simulink model "EVCS_model_v2"  (R2024b)
settings: Solver=VariableStepAuto  StartTime=0.0  StopTime=210  MaxStep=1e-3  RelTol=1e-2  AbsTol=1e-3
undefined symbols (not defined in the file or in its folder): FC, gcbh, Ion, Lithium, P, sps_rtmsupport, Ts
libraries: spsSeriesRLCBranchLib x40, spsIGBTDiodeLib x8, slpidlib x7, spsVoltageMeasurementLib x7, spsCurrentMeasurementLib x6, eeGeneralControl x4, spsMosfetLib x4, spsPWMGeneratorDCDCLib x3, spsAlphaBetaZerotodq0Lib x2, spsBatteryLib x2, spsDiodeLib x2, spsBreakerLib x1
(part 1 of 2)
settings Model: Creator=VidhiGupta  LastModifiedBy=akshat
settings RTWCC: GPUComputeCapability=3.5

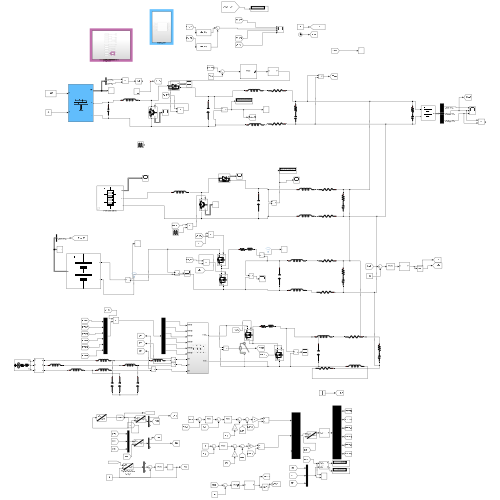
[thumbnail: Simulink's stored preview of the top-level diagram]
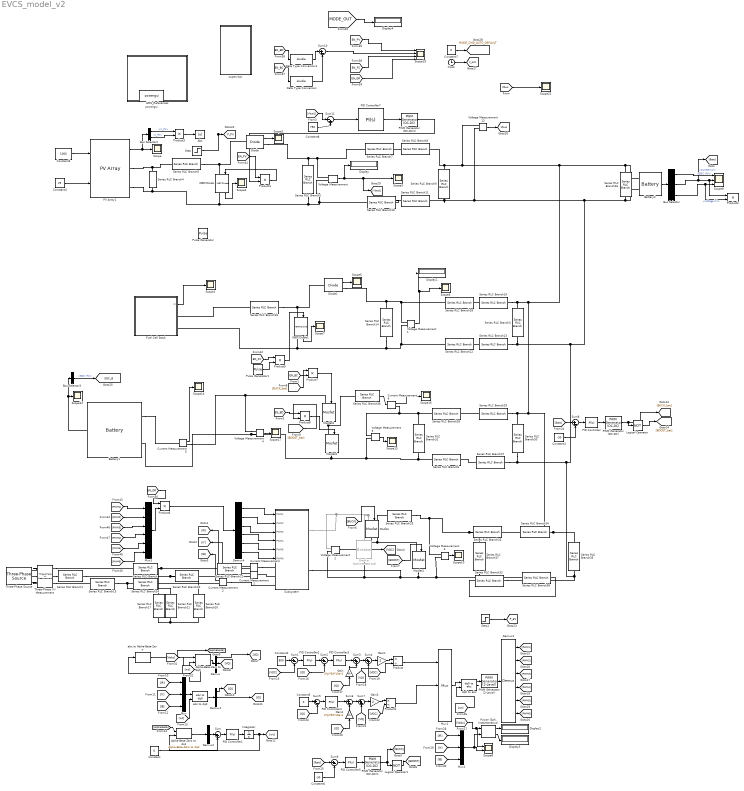
== system EVCS_model_v2 ==
  Abs : Abs  SaturateOnIntegerOverflow=off
  Alpha-Beta-Zero to dq0 : spsAlphaBetaZerotodq0Lib/Alpha-Beta-Zero to dq0  Alignment=90 degrees behind phase A axis
  Alpha-Beta-Zero to dq1 : spsAlphaBetaZerotodq0Lib/Alpha-Beta-Zero to dq0  Alignment=90 degrees behind phase A axis
  Battery1 : spsBatteryLib/Battery  BatType=Lithium-Ion  NomV=400  NomQ=250  SOC=60  Batt_Tr=30  PresetModel=on  MaxQ=250  MinV=300  FullV=465.5949  Dis_rate=108.6957  R=0.016  Normal_OP=226.087  expZone="[432.1543      12.28261]"
  Battery2 : spsBatteryLib/Battery  BatType=Lithium-Ion  NomV=400  NomQ=188  SOC=30  Batt_Tr=1  PresetModel=on  MaxQ=188  MinV=300  FullV=465.5949  Dis_rate=81.7391  R=0.021277  Normal_OP=170.0174  expZone="[432.1543      9.236522]"
  Breaker : spsBreakerLib/Breaker  Commented=on  InitialState=0  SwitchingTimes="[1/60  5/60]"  External=off  BreakerResistance=0.000001  SnubberResistance=1e6  SnubberCapacitance=inf  Measurements=None  MoreParameters=on  NoBreakLoop=off
  Bus Selector : BusSelector  OutputSignals=SOC (%),Current (A),Voltage (V)
  Bus Selector2 : BusSelector  OutputSignals=V_PV,I_PV
  Bus Selector3 : BusSelector  OutputSignals=SOC (%)
  Clock : Clock
  Constant : Constant  Value=0
  Constant1 : Constant  Value=-30
  Constant2 : Constant  Value=800
  Constant3 : Constant  Value=1000
  Constant4 : Constant  Value=25
  Constant5 : Constant  Value=0
  Constant6 : Constant  Value=-30
  Constant7 : Constant  Value=0
  Constant8 : Constant  Value=750
  Current Measurement{,1..2,5..6} (5 alike) : spsCurrentMeasurementLib/Current Measurement  PhasorSimulation=off  OutputType=Complex  PSBequivalent=0
  Data Type Conversion : DataTypeConversion  OutDataTypeStr=double  SaturateOnIntegerOverflow=off  RndMeth=Floor
  Data Type Conversion1 : DataTypeConversion  OutDataTypeStr=double  SaturateOnIntegerOverflow=off  RndMeth=Floor
  Demux : Demux  Outputs=3
  Demux1 : Demux  Outputs=3
  Demux2 : Demux  Outputs=3
  Demux3 : Demux  Outputs=6
  Demux4 : Demux  Outputs=6
  Diode : spsDiodeLib/Diode  Ron=0.001  Lon=0  Vf=0.8  IC=0  UseSnubber=0  Rs=500  Cs=250e-9  Measurements=on
  Diode1 : spsDiodeLib/Diode  Ron=0.001  Lon=0  Vf=0.8  IC=0  UseSnubber=0  Rs=500  Cs=250e-9  Measurements=on
  Display{,1..4} (5 alike) : Display
  EMS_References : Subsystem
  Fuel Cell Stack : Subsystem  AncestorBlock=sps_lib/Sources/Fuel Cell Stack  LoadFcn=sps_rtmsupport('LoadFcn',gcbh);  StartFcn=sps_rtmsupport('StartFcn',gcbh);  StopFcn=sps_rtmsupport('StopFcn',gcbh);  mask(Fuel Cell Stack){PresetModel=No (User-Defined), FcType=0, Detailed=Simplified, Eoc=P.FC.Eoc, NomVI=P.FC.NomVI, EndVI=P.FC.EndVI, Nc=P.FC.Nc, n=55, TOp=65, AirFr=2500, SuppPress=[3, 1.5], Comp=[99.95,21,1], SignX=off, SignY=off, FlowRateH2=off, FlowRateAir=off, SystemTemp=off, SystemPH2=off, SystemPAir=off, FCDyn=off, FC_tau=1, Peak_O2=80, V_Under=10}
      mask prompts: PresetModel "Preset model:"; FcType "Fuel Cell type:"; Detailed "Model detail Level:"; Eoc "Voltage at 0A and 1A [V_0(V), V_1(V)]"; NomVI "Nominal operating point [Inom(A), Vnom(V)]"; EndVI "Maximum operating point [Iend(A), Vend(V)]"; Nc "Number of cells"; n "Nominal stack efficiency (%)"; TOp "Operating temperature (Celsius)"; AirFr "Nominal Air flow rate (lpm)"; SuppPress "Nominal supply pressure [Fuel (atm), Air (atm)]"; Comp "Nominal composition (%) [H2 O2 H2O(Air)]"; SignX "Fuel  composition [x_H2(%)]"; SignY "Oxidant composition [y_O2(%)]"; FlowRateH2 "Fuel flow rate [FuelFr(lpm)]"; FlowRateAir "Air flow rate [AirFr(lpm)]"; SystemTemp "System Temperature [T(Kelvin)]"; SystemPH2 "Fuel supply pressure [Pfuel(bar)]"; SystemPAir "Air supply pressure [PAir(bar)]"; FCDyn "Specify Fuel Cell Dynamics?"; FC_tau "Fuel Cell response time (sec)"; Peak_O2 "Peak O2 utilization (%)"; V_Under "Voltage undershoot (V) @ peak O2 utilization"
      mask help:
      | Implements a generic hydrogen fuel cell model which allows the simulation for the following types of cells:
      | - Proton Exchange Membrane Fuel Cell (PEMFC)
      | - Solid Oxide Fuel Cell (SOFC)
      | - Alkaline Fuel Cell (AFC)
      mask init:
      | block = gcb;
      | %% DO NOT CHANGE THIS ORDER
      | FuelCellBlockCback(block,'Inputs')
      | [FC, WantBlockChoice, Ts] = FuelCellBlockInit(block,Eoc,NomVI,EndVI,Nc,n,TOp,AirFr,SuppPress,Comp,FlowRateH2,FlowRateAir);
      | powericon('SetInternalModels','set',block,WantBlockChoice);
      settings: LibrarySourceBlock=sps_lib/Sources/Fuel Cell Stack  CopyFcn=sps_rtmsupport('CopyFcn',gcbh);  DeleteFcn=sps_rtmsupport('DeleteFcn',gcbh);  UndoDeleteFcn=sps_rtmsupport('UndoDeleteFcn',gcbh);  ModelCloseFcn=sps_rtmsupport('ModelCloseFcn',gcbh);  PreSaveFcn=sps_rtmsupport('PreSaveFcn',gcbh);  PostSaveFcn=sps_rtmsupport('PostSaveFcn',gcbh);  NameChangeFcn=sps_rtmsupport('NameChangeFcn',gcbh);  PreCopyFcn=sps_rtmsupport('PreCopyFcn',gcbh);  OpenFcn=sps_rtmsupport('OpenFcn',gcbh, [1 2 3 13 14 15 16 17 18 19 20]);  CloseFcn=sps_rtmsupport('CloseFcn',gcbh);  PreDeleteFcn=sps_rtmsupport('PreDeleteFcn',gcbh);
      mask Help: helpview(psbhelp)
      mask TypeOptions PresetModel: No (User-Defined) | PEMFC - 1.26 kW - 24 Vdc | PEMFC - 6 kW - 45 Vdc | PEMFC - 50 kW - 625 Vdc | AFC - 2.4 kW - 48 Vdc | SOFC - 3 kW - 100 Vdc | SOFC - 25 kW - 630 Vdc
      mask Callback PresetModel: FuelCellBlockCback(gcb,'Preset')
      mask TypeOptions Detailed: Simplified | Detailed
      mask Callback Detailed: FuelCellBlockCback(gcb,'Visibilities')
      mask Callback FlowRateAir: FuelCellBlockCback(gcb,'Visibilities')
      mask Callback FCDyn: FuelCellBlockCback(gcb,'Visibilities')
      mask DialogControl ParameterTabVar0 Prompt: Parameters
      mask DialogControl plot_graph Prompt: Plot V_I characteristic
      mask DialogControl plot_graph Callback: FuelCellBlockCback(gcb,'PlotGraph');
      mask DialogControl ViewParam Prompt: View Cell parameters
      mask DialogControl ViewParam Callback: FuelCellBlockCback(gcb,'ViewParam');
      mask DialogControl ParameterTabVar01 Prompt: Signal variation
      mask DialogControl ParameterTabVar012 Prompt: Fuel Cell Dynamics
      mask Display: image(fullfile(matlabroot,'toolbox','physmod','powersys','library','sources','FuelCellStackBlockIcon.png'), [3,0,3,0,100,100]);
  Gain : Gain  Gain=2*pi*50*10e-3
  Gain1 : Gain  Gain=2
  Gain2 : Gain  Gain=2*pi*50*10e-3
  Gain3 : Gain  Gain=2
  IGBT/Diode : spsIGBTDiodeLib/IGBT//Diode  Ron=1e-3  Rs=1e5  Cs=inf  Measurements=on
  IGBT/Diode1 : spsIGBTDiodeLib/IGBT//Diode  Ron=1e-3  Rs=1e5  Cs=inf  Measurements=on
  Integrator : Integrator
  Logical Operator : Logic  Operator=NOT  AllPortsSameDT=off  OutDataTypeStr=boolean
  Logical Operator1 : Logic  Operator=NOT  AllPortsSameDT=off  OutDataTypeStr=boolean
  Mosfet{,1,3..4} (4 alike) : spsMosfetLib/Mosfet  Ron=0.001  Lon=0  Rd=1e-3  Vfd=0  IC=0  Rs=1e5  Cs=inf  Measurements=off
  Mux : Mux  Inputs=3
  Mux1 : Mux  Inputs=3
  Mux2 : Mux  Inputs=3
  Mux3 : Mux  Inputs=6
  PID Controller{,1..4} (5 alike) : slpidlib/PID Controller  Controller=PI  Form=Parallel  TimeDomain=Continuous-time  UseExternalTs=off  SampleTime=-1  IntegratorMethod=Forward Euler  FilterMethod=Forward Euler  ControllerParametersSource=internal  P=0.5  I=50  UseKiTs=off  D=0  UseExternalDerivativeSource=off  N=100  UseFilter=on  TunerSelectOption=Transfer Function Based (PID Tuner App)  InitialConditionSource=internal  InitialConditionForIntegrator=0  InitialConditionForFilter=0  DifferentiatorICPrevScaledInput=0  ExternalReset=none  TrackingMode=off  Kt=1  LimitOutput=off  SatLimitsSource=internal  UpperSaturationLimit=inf  LowerSaturationLimit=-inf  LinearizeAsGain=on  AntiWindupMode=none  Kb=1  LimitIntegrator=off  UpperIntegratorSaturationLimit=inf  LowerIntegratorSaturationLimit=-inf  POutMin=[]  POutMax=[]  IOutMin=[]  IOutMax=[]  DOutMin=[]  DOutMax=[]  NOutMin=[]  NOutMax=[]  SumOutMin=[]  SumOutMax=[]  SaturationOutMin=[]  SaturationOutMax=[]  PParamMin=[]  PParamMax=[]  IParamMin=[]  IParamMax=[]  DParamMin=[]  DParamMax=[]  NParamMin=[]  NParamMax=[]  KbParamMin=[]  KbParamMax=[]  KtParamMin=[]  KtParamMax=[]  KbOutMin=[]  KbOutMax=[]  KtOutMin=[]  KtOutMax=[]  IntegratorOutMin=[]  IntegratorOutMax=[]  FilterOutMin=[]  FilterOutMax=[]  SumI1OutMin=[]  SumI1OutMax=[]  SumI2OutMin=[]  SumI2OutMax=[]  SumI3OutMin=[]  SumI3OutMax=[]  SumI4OutMin=[]  SumI4OutMax=[]  SumDOutMin=[]  SumDOutMax=[]  DifferentiatorOutMin=[]  DifferentiatorOutMax=[]  FilterDiffOutCoefMin=[]  FilterDiffOutCoefMax=[]  ReciprocalOutMin=[]  ReciprocalOutMax=[]  SumDenOutMin=[]  SumDenOutMax=[]  SumNumOutMin=[]  SumNumOutMax=[]  DivideOutMin=[]  DivideOutMax=[]  UdiffTsProdOutMin=[]  UdiffTsProdOutMax=[]  NTsProdOutMin=[]  NTsProdOutMax=[]  UintegralTsProdOutMin=[]  UintegralTsProdOutMax=[]  UngainTsProdOutMin=[]  UngainTsProdOutMax=[]  ClampingZeroOutDataTypeStr=Inherit: Inherit via back propagation  ClampingZeroOutMin=[]  ClampingZeroOutMax=[]  FilterDenConstantOutDataTypeStr=Inherit: Inherit via back propagation  FilterDenConstantOutMin=[]  FilterDenConstantOutMax=[]  PCopyOutDataTypeStr=Inherit: Inherit via back propagation  PCopyOutMin=[]  PCopyOutMax=[]  NCopyOutDataTypeStr=Inherit: Inherit via back propagation  NCopyOutMin=[]  NCopyOutMax=[]  IntegratorContinuousStateAttributes=''  IntegratorStateMustResolveToSignalObject=off  IntegratorRTWStateStorageClass=Auto  FilterContinuousStateAttributes=''  FilterStateMustResolveToSignalObject=off  FilterRTWStateStorageClass=Auto  ParallelPVariant=InternalParameters  IdealPVariant=Disabled  IVariant=InternalParameters  DVariant=Disabled  IntegratorVariant=Continuous  SatVariant=Disabled  AWVariant=Passthrough  PCopyVariant=Disabled  TRVariant=Disabled  FdbkBlocksVariant=Forward  IdealPFdbkVariant=Disabled  SatFdbkVariant=Disabled  DerivativeFilterVariant=Disabled  NVariant=Disabled  NCopyVariant=Disabled_SignalSpec  FilterICVariant=Disabled  IntegratorICVariant=InternalICs  ExternalResetVariant=Disabled  TRSumVariant=Passthrough  SumFdbkVariant=Disabled  SumVariant=Sum_PI  TsampFilterVariant=InternalTs  TsampNgainVariant=Passthrough  TsampIntegralVariant=Disabled_SignalSpec  ExternalSaturationOutDataTypeStr=Inherit: Same as second input  DerivativeSourceVariant=Disabled  PreIntVariant=InternalPreInt
  PID Controller5 : slpidlib/PID Controller  Controller=PI  Form=Parallel  TimeDomain=Continuous-time  UseExternalTs=off  SampleTime=-1  IntegratorMethod=Forward Euler  FilterMethod=Forward Euler  ControllerParametersSource=internal  P=0.5  I=50  UseKiTs=off  D=0  UseExternalDerivativeSource=off  N=100  UseFilter=on  TunerSelectOption=Transfer Function Based (PID Tuner App)  InitialConditionSource=internal  InitialConditionForIntegrator=0  InitialConditionForFilter=0  DifferentiatorICPrevScaledInput=0  ExternalReset=none  TrackingMode=off  Kt=1  LimitOutput=on  SatLimitsSource=internal  UpperSaturationLimit=0.95  LowerSaturationLimit=0  LinearizeAsGain=on  AntiWindupMode=none  Kb=1  LimitIntegrator=off  UpperIntegratorSaturationLimit=inf  LowerIntegratorSaturationLimit=-inf  POutMin=[]  POutMax=[]  IOutMin=[]  IOutMax=[]  DOutMin=[]  DOutMax=[]  NOutMin=[]  NOutMax=[]  SumOutMin=[]  SumOutMax=[]  SaturationOutMin=[]  SaturationOutMax=[]  PParamMin=[]  PParamMax=[]  IParamMin=[]  IParamMax=[]  DParamMin=[]  DParamMax=[]  NParamMin=[]  NParamMax=[]  KbParamMin=[]  KbParamMax=[]  KtParamMin=[]  KtParamMax=[]  KbOutMin=[]  KbOutMax=[]  KtOutMin=[]  KtOutMax=[]  IntegratorOutMin=[]  IntegratorOutMax=[]  FilterOutMin=[]  FilterOutMax=[]  SumI1OutMin=[]  SumI1OutMax=[]  SumI2OutMin=[]  SumI2OutMax=[]  SumI3OutMin=[]  SumI3OutMax=[]  SumI4OutMin=[]  SumI4OutMax=[]  SumDOutMin=[]  SumDOutMax=[]  DifferentiatorOutMin=[]  DifferentiatorOutMax=[]  FilterDiffOutCoefMin=[]  FilterDiffOutCoefMax=[]  ReciprocalOutMin=[]  ReciprocalOutMax=[]  SumDenOutMin=[]  SumDenOutMax=[]  SumNumOutMin=[]  SumNumOutMax=[]  DivideOutMin=[]  DivideOutMax=[]  UdiffTsProdOutMin=[]  UdiffTsProdOutMax=[]  NTsProdOutMin=[]  NTsProdOutMax=[]  UintegralTsProdOutMin=[]  UintegralTsProdOutMax=[]  UngainTsProdOutMin=[]  UngainTsProdOutMax=[]  ClampingZeroOutDataTypeStr=Inherit: Inherit via back propagation  ClampingZeroOutMin=[]  ClampingZeroOutMax=[]  FilterDenConstantOutDataTypeStr=Inherit: Inherit via back propagation  FilterDenConstantOutMin=[]  FilterDenConstantOutMax=[]  PCopyOutDataTypeStr=Inherit: Inherit via back propagation  PCopyOutMin=[]  PCopyOutMax=[]  NCopyOutDataTypeStr=Inherit: Inherit via back propagation  NCopyOutMin=[]  NCopyOutMax=[]  IntegratorContinuousStateAttributes=''  IntegratorStateMustResolveToSignalObject=off  IntegratorRTWStateStorageClass=Auto  FilterContinuousStateAttributes=''  FilterStateMustResolveToSignalObject=off  FilterRTWStateStorageClass=Auto  ParallelPVariant=InternalParameters  IdealPVariant=Disabled  IVariant=InternalParameters  DVariant=Disabled  IntegratorVariant=Continuous  SatVariant=Enabled  AWVariant=Passthrough  PCopyVariant=Disabled  TRVariant=Disabled  FdbkBlocksVariant=Forward  IdealPFdbkVariant=Disabled  SatFdbkVariant=Disabled  DerivativeFilterVariant=Disabled  NVariant=Disabled  NCopyVariant=Disabled_SignalSpec  FilterICVariant=Disabled  IntegratorICVariant=InternalICs  ExternalResetVariant=Disabled  TRSumVariant=Passthrough  SumFdbkVariant=Disabled  SumVariant=Sum_PI  TsampFilterVariant=InternalTs  TsampNgainVariant=Passthrough  TsampIntegralVariant=Disabled_SignalSpec  ExternalSaturationOutDataTypeStr=Inherit: Same as second input  DerivativeSourceVariant=Disabled  PreIntVariant=InternalPreInt
  PID Controller7 : slpidlib/PID Controller  Controller=PI  Form=Parallel  TimeDomain=Continuous-time  UseExternalTs=off  SampleTime=-1  IntegratorMethod=Forward Euler  FilterMethod=Forward Euler  ControllerParametersSource=internal  P=0.01  I=0.5  UseKiTs=off  D=0  UseExternalDerivativeSource=off  N=100  UseFilter=on  TunerSelectOption=Transfer Function Based (PID Tuner App)  InitialConditionSource=internal  InitialConditionForIntegrator=00.4  InitialConditionForFilter=0  DifferentiatorICPrevScaledInput=0  ExternalReset=none  TrackingMode=off  Kt=1  LimitOutput=on  SatLimitsSource=internal  UpperSaturationLimit=0.95  LowerSaturationLimit=0.05  LinearizeAsGain=on  AntiWindupMode=none  Kb=1  LimitIntegrator=off  UpperIntegratorSaturationLimit=inf  LowerIntegratorSaturationLimit=-inf  POutMin=[]  POutMax=[]  IOutMin=[]  IOutMax=[]  DOutMin=[]  DOutMax=[]  NOutMin=[]  NOutMax=[]  SumOutMin=[]  SumOutMax=[]  SaturationOutMin=[]  SaturationOutMax=[]  PParamMin=[]  PParamMax=[]  IParamMin=[]  IParamMax=[]  DParamMin=[]  DParamMax=[]  NParamMin=[]  NParamMax=[]  KbParamMin=[]  KbParamMax=[]  KtParamMin=[]  KtParamMax=[]  KbOutMin=[]  KbOutMax=[]  KtOutMin=[]  KtOutMax=[]  IntegratorOutMin=[]  IntegratorOutMax=[]  FilterOutMin=[]  FilterOutMax=[]  SumI1OutMin=[]  SumI1OutMax=[]  SumI2OutMin=[]  SumI2OutMax=[]  SumI3OutMin=[]  SumI3OutMax=[]  SumI4OutMin=[]  SumI4OutMax=[]  SumDOutMin=[]  SumDOutMax=[]  DifferentiatorOutMin=[]  DifferentiatorOutMax=[]  FilterDiffOutCoefMin=[]  FilterDiffOutCoefMax=[]  ReciprocalOutMin=[]  ReciprocalOutMax=[]  SumDenOutMin=[]  SumDenOutMax=[]  SumNumOutMin=[]  SumNumOutMax=[]  DivideOutMin=[]  DivideOutMax=[]  UdiffTsProdOutMin=[]  UdiffTsProdOutMax=[]  NTsProdOutMin=[]  NTsProdOutMax=[]  UintegralTsProdOutMin=[]  UintegralTsProdOutMax=[]  UngainTsProdOutMin=[]  UngainTsProdOutMax=[]  ClampingZeroOutDataTypeStr=Inherit: Inherit via back propagation  ClampingZeroOutMin=[]  ClampingZeroOutMax=[]  FilterDenConstantOutDataTypeStr=Inherit: Inherit via back propagation  FilterDenConstantOutMin=[]  FilterDenConstantOutMax=[]  PCopyOutDataTypeStr=Inherit: Inherit via back propagation  PCopyOutMin=[]  PCopyOutMax=[]  NCopyOutDataTypeStr=Inherit: Inherit via back propagation  NCopyOutMin=[]  NCopyOutMax=[]  IntegratorContinuousStateAttributes=''  IntegratorStateMustResolveToSignalObject=off  IntegratorRTWStateStorageClass=Auto  FilterContinuousStateAttributes=''  FilterStateMustResolveToSignalObject=off  FilterRTWStateStorageClass=Auto  ParallelPVariant=InternalParameters  IdealPVariant=Disabled  IVariant=InternalParameters  DVariant=Disabled  IntegratorVariant=Continuous  SatVariant=Enabled  AWVariant=Passthrough  PCopyVariant=Disabled  TRVariant=Disabled  FdbkBlocksVariant=Forward  IdealPFdbkVariant=Disabled  SatFdbkVariant=Disabled  DerivativeFilterVariant=Disabled  NVariant=Disabled  NCopyVariant=Disabled_SignalSpec  FilterICVariant=Disabled  IntegratorICVariant=InternalICs  ExternalResetVariant=Disabled  TRSumVariant=Passthrough  SumFdbkVariant=Disabled  SumVariant=Sum_PI  TsampFilterVariant=InternalTs  TsampNgainVariant=Passthrough  TsampIntegralVariant=Disabled_SignalSpec  ExternalSaturationOutDataTypeStr=Inherit: Same as second input  DerivativeSourceVariant=Disabled  PreIntVariant=InternalPreInt
  PV Array1 : spsPVArrayLib/PV Array  Npar=12  Nser=10  PlotType=array @ 1000 W/m2 & specified temperatures  S_vec="[ 1000  500  100 ]"  Temp_C_vec="[ 45 25  ]"  ModuleName=Ablytek 6MN6A280  PlotWhenSelected=off  Pm=280.0896  Ncell=60  Voc=39.31  Isc=9.51  Vm=31.26  Im=8.96  beta_Voc_pc=-0.3137  alpha_Isc_pc=0.052103  beta_Voc=-0.12331  alpha_Isc=0.004955  IL=9.5578  I0=5.7114e-11  nI=0.98731  Rsh=279.2025  Rs=0.39513  RobustModel=off  RobustCellTemperature=313.3991  BAL=on  Tc=1e-6  Tfilter=5e-5
  PWM Generator (2-Level) : spsPWMGenerator2LevelLib/PWM Generator (2-Level)  ModulatorType=Three-phase bridge (6 pulses)  ModulatorMode=Unsynchronized  Fc=10000  Pc=90  nF=27  MinMax="[ -1  1 ]"  SamplingTechnique=Natural  ModulatingSignals=off  m=0.8  Freq=50  Phase=0  Ts=0  ShowCarrierOutport=off
  PWM Generator (DC-DC) : spsPWMGeneratorDCDCLib/PWM Generator (DC-DC)  Fsw=10000  Ts=0
  PWM Generator (DC-DC)1 : spsPWMGeneratorDCDCLib/PWM Generator (DC-DC)  Fsw=10000  Ts=0
  PWM Generator (DC-DC)2 : spsPWMGeneratorDCDCLib/PWM Generator (DC-DC)  Fsw=10000  Ts=0
  "Power (3ph, Instantaneous)" : spsPower3phInstantaneousLib/Power (3ph, Instantaneous)
  Product : Product  Inputs=*/
  Product1 : Product  Inputs=*/
  Product{2..8} (7 alike) : Product
  Pulse Generator : DiscretePulseGenerator  PulseType=Time based  Period=0.0001  PulseWidth=50
  Pulse Generator1 : DiscretePulseGenerator  PulseType=Time based  Period=0.0001  PulseWidth=50
  Scope{,1..7,10,12..14,16..17,22} (15 alike) : Scope
  Scope19 : Scope  NumInputPorts=4
  Scope8 : Scope  NumInputPorts=2
  Scope9 : Scope  NumInputPorts=3
  Series RLC Branch{,1,15,22..24} (6 alike) : spsSeriesRLCBranchLib/Series RLC Branch  LConnTagsString=__new0  RConnTagsString=__new0  BranchType=L  Resistance=1  Inductance=5e-3  SetiL0=off  InitialCurrent=0  Capacitance=1e-6  Setx0=off  InitialVoltage=0  Measurements=None
  Series RLC Branch{5..7,10,12,16,18,28,33,38} (10 alike) : spsSeriesRLCBranchLib/Series RLC Branch  LConnTagsString=__new0  RConnTagsString=__new0  BranchType=L  Resistance=5e-3  Inductance=0.001  SetiL0=off  InitialCurrent=0  Capacitance=1e-6  Setx0=off  InitialVoltage=0  Measurements=None
  Series RLC Branch{8,11,13,19,27,29,32,34} (8 alike) : spsSeriesRLCBranchLib/Series RLC Branch  LConnTagsString=__new0  RConnTagsString=__new0  BranchType=R  Resistance=100  Inductance=0.003  SetiL0=off  InitialCurrent=0  Capacitance=1e-6  Setx0=off  InitialVoltage=0  Measurements=None
  Series RLC Branch14 : spsSeriesRLCBranchLib/Series RLC Branch  LConnTagsString=__new0  RConnTagsString=__new0  BranchType=C  Resistance=5e-3  Inductance=0.003  SetiL0=off  InitialCurrent=0  Capacitance=0.0047  Setx0=off  InitialVoltage=0  Measurements=None
  Series RLC Branch17 : spsSeriesRLCBranchLib/Series RLC Branch  LConnTagsString=__new0  RConnTagsString=__new0  BranchType=C  Resistance=1  Inductance=5e-3  SetiL0=off  InitialCurrent=0  Capacitance=30e-6  Setx0=off  InitialVoltage=0  Measurements=None
  Series RLC Branch2 : spsSeriesRLCBranchLib/Series RLC Branch  LConnTagsString=__new0  RConnTagsString=__new0  BranchType=C  Resistance=5e-3  Inductance=0.003  SetiL0=off  InitialCurrent=0  Capacitance=0.0047  Setx0=off  InitialVoltage=0  Measurements=None
  Series RLC Branch20 : spsSeriesRLCBranchLib/Series RLC Branch  LConnTagsString=__new0  RConnTagsString=__new0  BranchType=C  Resistance=1  Inductance=5e-3  SetiL0=off  InitialCurrent=0  Capacitance=30e-6  Setx0=off  InitialVoltage=0  Measurements=None
  Series RLC Branch21 : spsSeriesRLCBranchLib/Series RLC Branch  LConnTagsString=__new0  RConnTagsString=__new0  BranchType=C  Resistance=1  Inductance=5e-3  SetiL0=off  InitialCurrent=0  Capacitance=30e-6  Setx0=off  InitialVoltage=0  Measurements=None
  Series RLC Branch25 : spsSeriesRLCBranchLib/Series RLC Branch  LConnTagsString=__new0  RConnTagsString=__new0  BranchType=RL  Resistance=0.0001  Inductance=20e-3  SetiL0=off  InitialCurrent=0  Capacitance=1e-6  Setx0=off  InitialVoltage=0  Measurements=None
  Series RLC Branch26 : spsSeriesRLCBranchLib/Series RLC Branch  LConnTagsString=__new0  RConnTagsString=__new0  BranchType=RC  Resistance=0.0001  Inductance=20e-3  SetiL0=off  InitialCurrent=0  Capacitance=0.625e-6  Setx0=off  InitialVoltage=0  Measurements=None
  Series RLC Branch3 : spsSeriesRLCBranchLib/Series RLC Branch  LConnTagsString=__new0  RConnTagsString=__new0  BranchType=RC  Resistance=1e-3  Inductance=0.003  SetiL0=off  InitialCurrent=0  Capacitance=0.0047  Setx0=off  InitialVoltage=0  Measurements=None
  Series RLC Branch30 : spsSeriesRLCBranchLib/Series RLC Branch  LConnTagsString=__new0  RConnTagsString=__new0  BranchType=RC  Resistance=1e-3  Inductance=0.003  SetiL0=off  InitialCurrent=0  Capacitance=0.0047  Setx0=off  InitialVoltage=0  Measurements=None
  Series RLC Branch31 : spsSeriesRLCBranchLib/Series RLC Branch  LConnTagsString=__new0  RConnTagsString=__new0  BranchType=C  Resistance=5e-3  Inductance=0.003  SetiL0=off  InitialCurrent=0  Capacitance=0.0047  Setx0=off  InitialVoltage=0  Measurements=None
  Series RLC Branch35 : spsSeriesRLCBranchLib/Series RLC Branch  LConnTagsString=__new0  RConnTagsString=__new0  BranchType=RC  Resistance=1e-3  Inductance=0.003  SetiL0=off  InitialCurrent=0  Capacitance=0.0001  Setx0=off  InitialVoltage=0  Measurements=None
  Series RLC Branch36 : spsSeriesRLCBranchLib/Series RLC Branch  LConnTagsString=__new0  RConnTagsString=__new0  BranchType=RL  Resistance=0.0001  Inductance=50e-2  SetiL0=off  InitialCurrent=0  Capacitance=1e-6  Setx0=off  InitialVoltage=0  Measurements=None
  Series RLC Branch37 : spsSeriesRLCBranchLib/Series RLC Branch  LConnTagsString=__new0  RConnTagsString=__new0  BranchType=C  Resistance=5e-3  Inductance=0.003  SetiL0=off  InitialCurrent=0  Capacitance=0.0001  Setx0=off  InitialVoltage=0  Measurements=None
  Series RLC Branch4 : spsSeriesRLCBranchLib/Series RLC Branch  LConnTagsString=__new0  RConnTagsString=__new0  BranchType=C  Resistance=5e-3  Inductance=0.003  SetiL0=off  InitialCurrent=0  Capacitance=0.0001  Setx0=off  InitialVoltage=0  Measurements=None
  Series RLC Branch9 : spsSeriesRLCBranchLib/Series RLC Branch  LConnTagsString=__new0  RConnTagsString=__new0  BranchType=RC  Resistance=1e-3  Inductance=0.003  SetiL0=off  InitialCurrent=0  Capacitance=0.0001  Setx0=off  InitialVoltage=0  Measurements=None
  Step : Step  Time=5  Before=30000  After=0  SampleTime=0
  Step1 : Step  Time=10  Before=5000  After=0  SampleTime=0
  Subsystem : Subsystem
  Sum : Sum  Inputs=|-+
  Sum{1..2,5..6,8..10} (7 alike) : Sum  Inputs=|+-
  Sum11 : Sum  Inputs=|-+
  Sum3 : Sum  Inputs=|++
  Sum4 : Sum  Inputs=|++
  Sum7 : Sum  Inputs=|++
  Three-Phase V-I Measurement : spsThreePhaseVIMeasurementLib/Three-Phase V-I Measurement  VoltageMeasurement=phase-to-ground  SetLabelV=on  LabelV=Vabc  Vpu=off  VpuLL=off  CurrentMeasurement=no  SetLabelI=off  LabelI=Iabc  Ipu=off  Pbase=100e6  Vbase=500e3  OutputType=Complex  PhasorSimulation=off  PSBequivalent=0
  Three-Phase Source : spsThreePhaseSourceLib/Three-Phase Source  InternalConnection=Yg  VoltagePhases=off  Voltage=415  PhaseAngle=0  Voltage_phases=[239.600361713695 239.600361713695 239.600361713695]  PhaseAngles_phases=[0 -120 120]  Frequency=50  NonIdealSource=on  SpecifyImpedance=off  Resistance=0.8929e-3  Inductance=16.58e-9  ShortCircuitLevel=100000000  BaseVoltage=415  XRratio=7  BusType=swing  Pref=10e3  Qref=0  Prefabc=[10e3, 10e3, 10e3]  Qrefabc=[0, 0, 0]  Qmin=-inf  Qmax=inf
  Voltage Measurement{,1..2,4..6,12} (7 alike) : spsVoltageMeasurementLib/Voltage Measurement  PhasorSimulation=off  OutputType=Complex  PSBequivalent=0
  abc to Alpha-Beta-Zero : spsabctoAlphaBetaZeroLib/abc to Alpha-Beta-Zero
  abc to dq0 : spsabctodq0Lib/abc to dq0  Alignment=90 degrees behind phase A axis
  dq0 to abc : spsdq0toabcLib/dq0 to abc  Alignment=90 degrees behind phase A axis
  powergui : sps_lib/powergui  Priority=1  SimulationMode=Discrete  SampleTime=5e-06  frequency=60  Iterations=50  frequencyindice=0  Pbase=100e6  ErrMax=1e-4  UnitsV=kV  UnitsW=MW  buscounter=0  FunctionMessages=off  echomessages=off  EnableUseOfTLC=off  CurrentSourceSwitches=off  DisableSnubberDevices=off  DisableRonSwitches=off  DisableVfSwitches=off  DisplayEquations=off  AutomaticDiscreteSolvers=off  SolverType=Tustin/Backward Euler (TBE)  Interpol=off  ExternalGateDelay=off  methode=off  Ts=100  x0status=blocks  SPID=on  SwTol=0  HookPort=off  NonlinearTolerance=1e-4  nMaxIteration=100  ContinueOnMaxIteration=off  RestoreLinks=warning  ResistiveCurrentMeasurement=off  Frange=[0:2:500]  Ylog=off  Xlog=on  ShowGrid=off  save=off  variable=ZData  structure=0  ZoomFFT=off  StartTime=0.0  cycles=1  DisplayStyle=1  fundamental=60  FreqAxis=off  MaxFrequency=1000  frequencyindicesteady=1  RmsSteady=1  display=off
  supervisor : Subsystem
  tag scope: MODE_CMD_AUTO_DEFAULT=global, P_EV=global, P_PV=global, SOC_B=global, Vbus=global, t_sim=global
  wires:
  Constant4/1 -> PV Array1/2
  Constant3/1 -> PV Array1/1
  PV Array1/1 -> Bus Selector2/1, Scope/1
  Fuel Cell Stack/1(m) -> Scope1/1
  Voltage Measurement/1 -> [Vbus1], Scope3/1, Display/1
  Diode/1 -> Scope2/1
  IGBT/Diode/1 -> Scope4/1
  Diode1/1 -> Scope5/1
  Pulse Generator1/1 -> Product5/2
  IGBT/Diode1/1 -> Scope7/1
  Voltage Measurement1/1 -> Scope6/1, Display1/1
  Bus Selector/2 -> [Ibat], Product2/1, Scope9/2  "<Current (A)>"
  Battery2/1 -> Bus Selector/1
  Bus Selector/1 -> Scope9/1  "<SOC (%)>"
  Bus Selector/3 -> Product2/2, Scope9/3  "<Voltage (V)>"
  Current Measurement5/1 -> Scope14/1
  Logical Operator/1 -> [BOOST_bat]
  Constant1/1 -> Sum8/2
  PID Controller/1 -> PWM Generator (DC-DC)/1
  Voltage Measurement5/1 -> Scope13/1
  Current Measurement6/1 -> Scope16/1
  [Ibat] -> Sum8/1
  Sum8/1 -> PID Controller/1
  Voltage Measurement4/1 -> Scope17/1
  [BUCK_bat] -> Product7/2
  PWM Generator (DC-DC)/1 -> Logical Operator/1, [BUCK_bat]
  [BOOST_bat] -> Product8/2
  Battery1/1 -> Bus Selector3/1, Scope12/1
  Voltage Measurement6/1 -> Scope10/1
  [BUCK] -> Mosfet/1
  Current Measurement1/1 -> [IY]
  Voltage Measurement2/1 -> [VDC]
  [BOOST] -> Mosfet1/1
  Current Measurement/1 -> [IR]
  Current Measurement2/1 -> [IB]
  Logical Operator1/1 -> [BOOST]
  Product/1 -> Mux1/1
  [wt] -> dq0 to abc/2
  [VDC] -> Product/2
  Gain2/1 -> Sum6/2
  PID Controller5/1 -> PWM Generator (DC-DC)1/1
  Sum3/1 -> Sum4/1
  PID Controller4/1 -> Sum6/1
  [ID] -> Gain2/1
  [Ibat] -> Sum9/1
  PID Controller3/1 -> Sum3/1
  Sum9/1 -> PID Controller5/1
  PID Controller2/1 -> Sum2/1
  abc to Alpha-Beta-Zero/1 -> [alphabeta], Alpha-Beta-Zero to dq0/1
  [VQ] -> Sum7/2
  Constant5/1 -> Sum5/1
  [VD] -> Sum4/2
  Sum2/1 -> PID Controller3/1
  Gain1/1 -> Product/1
  Sum4/1 -> Gain1/1
  Mux/1 -> abc to dq0/1
  Integrator/1 -> [wt], Alpha-Beta-Zero to dq1/2
  Demux/1 -> [VD]
  Demux/2 -> [VQ]
  [IR] -> Mux/1
  abc to dq0/1 -> Demux1/1
  Sum6/1 -> Sum7/1
  [wt] -> Alpha-Beta-Zero to dq0/2
  "Power (3ph, Instantaneous)"/1 -> Display2/1
  [IQ] -> Gain/1
  [Vabc] -> abc to Alpha-Beta-Zero/1
  [IY] -> Mux/2
  [wt] -> abc to dq0/2
  "Power (3ph, Instantaneous)"/2 -> Display3/1
  [VDC] -> Product1/2
  [IB] -> Mux2/3
  Demux1/1 -> [ID]
  [alphabeta] -> Alpha-Beta-Zero to dq1/1
  PWM Generator (2-Level)/1 -> Demux3/1
  Demux3/3 -> [PWM3]
  Constant2/1 -> Sum1/1
  Mux2/1 -> "Power (3ph, Instantaneous)"/2, Scope8/2
  Demux2/2 -> Sum/1
  Demux3/6 -> [PWM6]
  PWM Generator (DC-DC)1/1 -> Logical Operator1/1, [BUCK]
  Demux1/2 -> [IQ]
  Constant/1 -> Sum/2
  Sum/1 -> PID Controller1/1
  Alpha-Beta-Zero to dq0/1 -> Demux/1
  [ID] -> Sum2/2
  [IY] -> Mux2/2
  Gain/1 -> Sum3/2
  [IB] -> Mux/3
  Sum7/1 -> Gain3/1
  PID Controller1/1 -> Integrator/1
  [Vabc] -> Scope8/1, "Power (3ph, Instantaneous)"/1
  Demux3/2 -> [PWM2]
  Alpha-Beta-Zero to dq1/1 -> Demux2/1
  Constant6/1 -> Sum9/2
  Sum1/1 -> PID Controller2/1
  [IQ] -> Sum5/2
  Product1/1 -> Mux1/2
  Demux3/4 -> [PWM4]
  [VDC] -> Sum1/2
  Gain3/1 -> Product1/1
  Demux3/1 -> [PWM1]
  Demux3/5 -> [PWM5]
  Sum5/1 -> PID Controller4/1
  [IR] -> Mux2/1
  Mux1/1 -> dq0 to abc/1
  dq0 to abc/1 -> PWM Generator (2-Level)/1
  Bus Selector2/1 -> Product3/1  "<V_PV>"
  Bus Selector2/2 -> Product3/2  "<I_PV>"
  Bus Selector3/1 -> [SOC_B]  "<SOC (%)>"
  Voltage Measurement12/1 -> [Vbus]
  Clock/1 -> [t_sim]
  Constant7/1 -> [MODE_CMD_AUTO_DEFAULT]
  [EN_FC] -> Scope19/3
  [EN_BC] -> Data Type Conversion/1
  [EN_BD] -> Data Type Conversion1/1
  [EN_GR] -> Scope19/4
  [EN_PV] -> Scope19/1
  Sum10/1 -> Scope19/2
  [MODE_OUT] -> Display4/1
  Data Type Conversion/1 -> Sum10/2
  Data Type Conversion1/1 -> Sum10/1
  Product3/1 -> Abs/1
  Step/1 -> [P_PV]
  [EN_PV] -> Product4/1
  Product4/1 -> IGBT/Diode/1
  [EN_FC] -> Product5/1
  Product5/1 -> IGBT/Diode1/1
  [PWM1] -> Mux3/1
  [PWM2] -> Mux3/2
  [PWM3] -> Mux3/3
  [PWM4] -> Mux3/4
  [PWM5] -> Mux3/5
  [PWM6] -> Mux3/6
  Mux3/1 -> Product6/2
  [EN_GR] -> Product6/1
  Product6/1 -> Demux4/1
  Demux4/1 -> Subsystem/1(PWM1)
  Demux4/2 -> Subsystem/2(PWM2)
  Demux4/3 -> Subsystem/3(PWM3)
  Demux4/4 -> Subsystem/4(PWM4)
  Demux4/5 -> Subsystem/5(PWM5)
  Demux4/6 -> Subsystem/6(PWM6)
  [Vbus] -> Scope22/1
  [EN_BC] -> Product7/1
  Product7/1 -> Mosfet3/1
  Product8/1 -> Mosfet4/1
  [EN_BD] -> Product8/1
  Step1/1 -> [P_EV]
  [Vbus1] -> Sum11/1
  Constant8/1 -> Sum11/2
  Sum11/1 -> PID Controller7/1
  PID Controller7/1 -> PWM Generator (DC-DC)2/1
  PWM Generator (DC-DC)2/1 -> Product4/2
  connections:
  PV Array1/RConn1 -- Series RLC Branch4/LConn1 -- Series RLC Branch5/LConn1
  Series RLC Branch5/RConn1 -- Diode/LConn1 -- IGBT/Diode/LConn1
  IGBT/Diode/RConn1 -- Voltage Measurement/LConn2 -- Series RLC Branch10/LConn1 -- Series RLC Branch2/RConn1 -- PV Array1/RConn2 -- Series RLC Branch4/RConn1
  Diode/RConn1 -- Series RLC Branch7/LConn1 -- Voltage Measurement/LConn1 -- Series RLC Branch2/LConn1
  Series RLC Branch8/RConn1 -- Series RLC Branch7/RConn1
  Series RLC Branch11/RConn1 -- Series RLC Branch10/RConn1
  Voltage Measurement1/LConn2 -- Series RLC Branch12/LConn1 -- Series RLC Branch14/RConn1 -- Fuel Cell Stack/RConn2 -- IGBT/Diode1/RConn1
  Series RLC Branch16/RConn1 -- IGBT/Diode1/LConn1 -- Diode1/LConn1
  Diode1/RConn1 -- Series RLC Branch18/LConn1 -- Voltage Measurement1/LConn1 -- Series RLC Branch14/LConn1
  Series RLC Branch19/RConn1 -- Series RLC Branch18/RConn1
  Series RLC Branch13/RConn1 -- Series RLC Branch12/RConn1
  Series RLC Branch16/LConn1 -- Fuel Cell Stack/RConn1
  Mosfet3/RConn1 -- Mosfet4/LConn1 -- Series RLC Branch36/LConn1
  Series RLC Branch38/LConn1 -- Breaker/RConn1 -- Voltage Measurement2/LConn2 -- Subsystem/RConn2 -- Mosfet1/RConn1 -- Voltage Measurement6/LConn2 -- Series RLC Branch37/RConn1
  Voltage Measurement4/LConn1 -- Current Measurement5/RConn1 -- Mosfet3/LConn1
  Battery1/LConn1 -- Current Measurement5/LConn1
  Series RLC Branch36/RConn1 -- Current Measurement6/LConn1
  Series RLC Branch22/LConn1 -- Series RLC Branch17/LConn1 -- Series RLC Branch/RConn1
  Series RLC Branch15/RConn1 -- Series RLC Branch24/LConn1 -- Series RLC Branch21/LConn1
  Series RLC Branch20/RConn1 -- Series RLC Branch17/RConn1 -- Series RLC Branch21/RConn1
  Series RLC Branch34/LConn1 -- Series RLC Branch35/LConn1 -- Series RLC Branch30/LConn1 -- Series RLC Branch29/LConn1 -- Series RLC Branch3/LConn1 -- Series RLC Branch19/LConn1 -- Series RLC Branch26/LConn1 -- Battery2/LConn1 -- Voltage Measurement12/LConn1 -- Series RLC Branch9/LConn1 -- Series RLC Branch8/LConn1
  Series RLC Branch1/RConn1 -- Series RLC Branch20/LConn1 -- Series RLC Branch23/LConn1
  Mosfet1/LConn1 -- Series RLC Branch25/LConn1 -- Mosfet/RConn1
  Breaker/LConn1 -- Subsystem/RConn1 -- Voltage Measurement2/LConn1 -- Mosfet/LConn1
  Current Measurement2/RConn1 -- Series RLC Branch24/RConn1
  Current Measurement1/RConn1 -- Series RLC Branch23/RConn1
  Three-Phase Source/RConn3 -- Three-Phase V-I Measurement/LConn3
  Three-Phase V-I Measurement/RConn3 -- Series RLC Branch15/LConn1
  Three-Phase V-I Measurement/RConn1 -- Series RLC Branch/LConn1
  Subsystem/LConn2 -- Current Measurement1/LConn1
  Current Measurement/RConn1 -- Series RLC Branch22/RConn1
  Three-Phase Source/RConn2 -- Three-Phase V-I Measurement/LConn2
  Current Measurement/LConn1 -- Subsystem/LConn1
  Current Measurement2/LConn1 -- Subsystem/LConn3
  Three-Phase V-I Measurement/RConn2 -- Series RLC Branch1/LConn1
  Three-Phase V-I Measurement/LConn1 -- Three-Phase Source/RConn1
  Series RLC Branch27/RConn1 -- Series RLC Branch6/RConn1
  Series RLC Branch29/RConn1 -- Series RLC Branch28/RConn1
  Current Measurement6/RConn1 -- Series RLC Branch31/LConn1 -- Series RLC Branch28/LConn1 -- Voltage Measurement5/LConn1
  Mosfet4/RConn1 -- Series RLC Branch31/RConn1 -- Series RLC Branch6/LConn1 -- Voltage Measurement5/LConn2 -- Battery1/LConn2 -- Voltage Measurement4/LConn2
  Series RLC Branch32/RConn1 -- Series RLC Branch38/RConn1
  Series RLC Branch34/RConn1 -- Series RLC Branch33/RConn1
  Series RLC Branch37/LConn1 -- Series RLC Branch25/RConn1 -- Voltage Measurement6/LConn1 -- Series RLC Branch33/LConn1
  Series RLC Branch35/RConn1 -- Series RLC Branch32/LConn1 -- Series RLC Branch3/RConn1 -- Series RLC Branch13/LConn1 -- Series RLC Branch26/RConn1 -- Battery2/LConn2 -- Voltage Measurement12/LConn2 -- Series RLC Branch11/LConn1 -- Series RLC Branch9/RConn1 -- Series RLC Branch27/LConn1 -- Series RLC Branch30/RConn1

== system EVCS_model_v2/EMS_References ==
  MODE_CMD : FromWorkspace  VariableName=MODE_CMD  SampleTime=-1  Interpolate=off  OutputAfterFinalValue=Holding final value
  P_EV : FromWorkspace  VariableName=P_EV  SampleTime=-1  Interpolate=off  OutputAfterFinalValue=Holding final value
  P_batt_set : FromWorkspace  VariableName=P_batt_set  SampleTime=-1  Interpolate=off  OutputAfterFinalValue=Holding final value
  P_grid_set : FromWorkspace  VariableName=P_grid_set  SampleTime=-1  Interpolate=off  OutputAfterFinalValue=Holding final value
  P_h2_set : FromWorkspace  VariableName=P_h2_set  SampleTime=-1  Interpolate=off  OutputAfterFinalValue=Holding final value
  P_load : FromWorkspace  VariableName=P_load  SampleTime=-1  Interpolate=off  OutputAfterFinalValue=Holding final value
  P_solar_set : FromWorkspace  VariableName=P_solar_set  SampleTime=-1  Interpolate=off  OutputAfterFinalValue=Holding final value
  Scope_Enables : Scope  NumInputPorts=4
  Scope_LoadRef : Scope
  Scope_Mode : Scope
  Scope_Setpoints : Scope  NumInputPorts=4
  en_batt : FromWorkspace  VariableName=en_batt  SampleTime=-1  Interpolate=off  OutputAfterFinalValue=Holding final value
  en_grid : FromWorkspace  VariableName=en_grid  SampleTime=-1  Interpolate=off  OutputAfterFinalValue=Holding final value
  en_h2 : FromWorkspace  VariableName=en_h2  SampleTime=-1  Interpolate=off  OutputAfterFinalValue=Holding final value
  en_solar : FromWorkspace  VariableName=en_solar  SampleTime=-1  Interpolate=off  OutputAfterFinalValue=Holding final value
  tag scope: MODE_CMD=global, P_EV_REF=global
  wires:
  MODE_CMD/1 -> [MODE_CMD], Scope_Mode/1
  P_EV/1 -> [P_EV_REF]
  P_load/1 -> Scope_LoadRef/1
  P_solar_set/1 -> Scope_Setpoints/1
  P_batt_set/1 -> Scope_Setpoints/2
  P_h2_set/1 -> Scope_Setpoints/3
  P_grid_set/1 -> Scope_Setpoints/4
  en_solar/1 -> Scope_Enables/1
  en_batt/1 -> Scope_Enables/2
  en_h2/1 -> Scope_Enables/3
  en_grid/1 -> Scope_Enables/4

== system EVCS_model_v2/Fuel Cell Stack ==
  AirFr : Constant  Value=FC.AirFr
  Controlled Voltage Source : spsControlledVoltageSourceLib/Controlled Voltage Source  Initialize=on  Source_Type=AC  Amplitude=0  Phase=0  Frequency=0  Measurements=None
  Current Measurement : spsCurrentMeasurementLib/Current Measurement  PhasorSimulation=off  OutputType=Complex  PSBequivalent=0
  FuelFr : Constant  Value=FC.FuelFr
  Model : Subsystem  Variant=on  VariantControlMode=label  LabelModeActiveChoice=Discrete/Simplified
      settings: AttributesFormatString=%<BlockChoice>
  PAir : Constant  Value=FC.PAir
  Pfuel : Constant  Value=FC.Pf
  Saturation : Saturate  UpperLimit=inf  LowerLimit=0  LinearizeAsGain=off
  T : Constant  Value=FC.Tnom
  x_H2 : Constant  Value=FC.x*100
  y_O2 : Constant  Value=FC.y*100
  + : PMIOPort  Side=Right
  - : PMIOPort  Port=2  Side=Right
  m : Outport  VectorParamsAs1DForOutWhenUnconnected=off
  wires:
  Saturation/1 -> Model/1(stackCurrent)
  [stackCurrent] -> Saturation/1  "stackCurrent"
  x_H2/1 -> Model/2(FuelVolumeFraction)
  y_O2/1 -> Model/3(OxygenVolumeFraction)
  FuelFr/1 -> Model/4(FuelVolumetricFlowRate)
  AirFr/1 -> Model/5(AirVolumetricFlowRate)
  T/1 -> Model/6(Temperature)
  Pfuel/1 -> Model/7(FuelSupplyPressure)
  PAir/1 -> Model/8(AirSupplyPressure)
  Current Measurement/1 -> [stackCurrent]
  Model/2(m) -> m/1
  Model/1(Voltage) -> Controlled Voltage Source/1
  connections:
  Controlled Voltage Source/LConn1 -- -/RConn1
  Controlled Voltage Source/RConn1 -- Current Measurement/LConn1
  +/RConn1 -- Current Measurement/RConn1

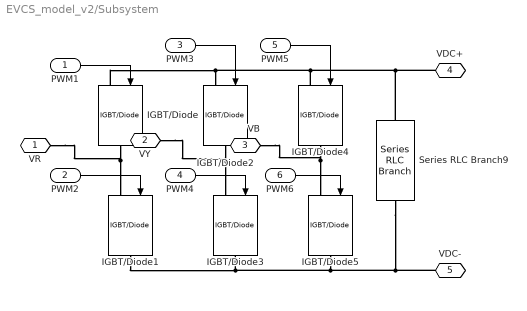
== system EVCS_model_v2/Subsystem ==
  PWM1 : Inport
  PWM2 : Inport  Port=2
  PWM3 : Inport  Port=3
  PWM4 : Inport  Port=4
  PWM5 : Inport  Port=5
  PWM6 : Inport  Port=6
  IGBT/Diode{,1..5} (6 alike) : spsIGBTDiodeLib/IGBT//Diode  Ron=1e-3  Rs=1e5  Cs=inf  Measurements=off
  Series RLC Branch9 : spsSeriesRLCBranchLib/Series RLC Branch  LConnTagsString=__new0  RConnTagsString=__new0  BranchType=RC  Resistance=1e-3  Inductance=1e-3  SetiL0=off  InitialCurrent=0  Capacitance=5600e-6  Setx0=on  InitialVoltage=800  Measurements=None
  VR : PMIOPort  Side=Left
  VY : PMIOPort  Port=2  Side=Left
  VB : PMIOPort  Port=3  Side=Left
  VDC+ : PMIOPort  Port=4  Side=Right
  VDC- : PMIOPort  Port=5  Side=Right
  wires:
  PWM5/1 -> IGBT/Diode4/1
  PWM4/1 -> IGBT/Diode3/1
  PWM2/1 -> IGBT/Diode1/1
  PWM1/1 -> IGBT/Diode/1
  PWM3/1 -> IGBT/Diode2/1
  PWM6/1 -> IGBT/Diode5/1
  connections:
  IGBT/Diode/RConn1 -- VR/RConn1 -- IGBT/Diode1/LConn1
  IGBT/Diode1/RConn1 -- VDC-/RConn1 -- Series RLC Branch9/RConn1 -- IGBT/Diode5/RConn1 -- IGBT/Diode3/RConn1
  IGBT/Diode4/RConn1 -- VB/RConn1 -- IGBT/Diode5/LConn1
  IGBT/Diode/LConn1 -- VDC+/RConn1 -- Series RLC Branch9/LConn1 -- IGBT/Diode4/LConn1 -- IGBT/Diode2/LConn1
  IGBT/Diode2/RConn1 -- VY/RConn1 -- IGBT/Diode3/LConn1

== system EVCS_model_v2/supervisor ==
  MATLAB Function : MATLAB Function  TreatAsAtomicUnit=on  SystemSampleTime=0.01
  tag scope: EN_BC=global, EN_BD=global, EN_FC=global, EN_GR=global, EN_PV=global, MODE_OUT=global
  wires:
  [P_EV_REF] -> MATLAB Function/1(P_EV_demand)
  [P_PV] -> MATLAB Function/2(P_PV_avail)
  [SOC_B] -> MATLAB Function/3(SOC_BESS)
  [Vbus] -> MATLAB Function/4(V_bus)
  [t_sim] -> MATLAB Function/5(t)
  [MODE_CMD] -> MATLAB Function/6(mode_cmd)
  MATLAB Function/1(en_PV) -> [EN_PV]
  MATLAB Function/2(en_BESS_dis) -> [EN_BD]
  MATLAB Function/3(en_BESS_chg) -> [EN_BC]
  MATLAB Function/4(en_FC) -> [EN_FC]
  MATLAB Function/5(en_GRID) -> [EN_GR]
  MATLAB Function/6(mode) -> [MODE_OUT]

== system EVCS_model_v2/Fuel Cell Stack/Model ==
  stackCurrent : Inport
  FuelVolumeFraction : Inport  Port=2
  OxygenVolumeFraction : Inport  Port=3
  FuelVolumetricFlowRate : Inport  Port=4
  AirVolumetricFlowRate : Inport  Port=5
  Temperature : Inport  Port=6
  FuelSupplyPressure : Inport  Port=7
  AirSupplyPressure : Inport  Port=8
  Continuous/Detailed : Subsystem  VariantControl=Continuous/Detailed
  Continuous/Simplified : Subsystem  VariantControl=Continuous/Simplified
  Discrete/Detailed : Subsystem  VariantControl=Discrete/Detailed
  Discrete/Simplified : Subsystem  VariantControl=Discrete/Simplified
  Voltage : Outport  VectorParamsAs1DForOutWhenUnconnected=off
  m : Outport  Port=2  VectorParamsAs1DForOutWhenUnconnected=off

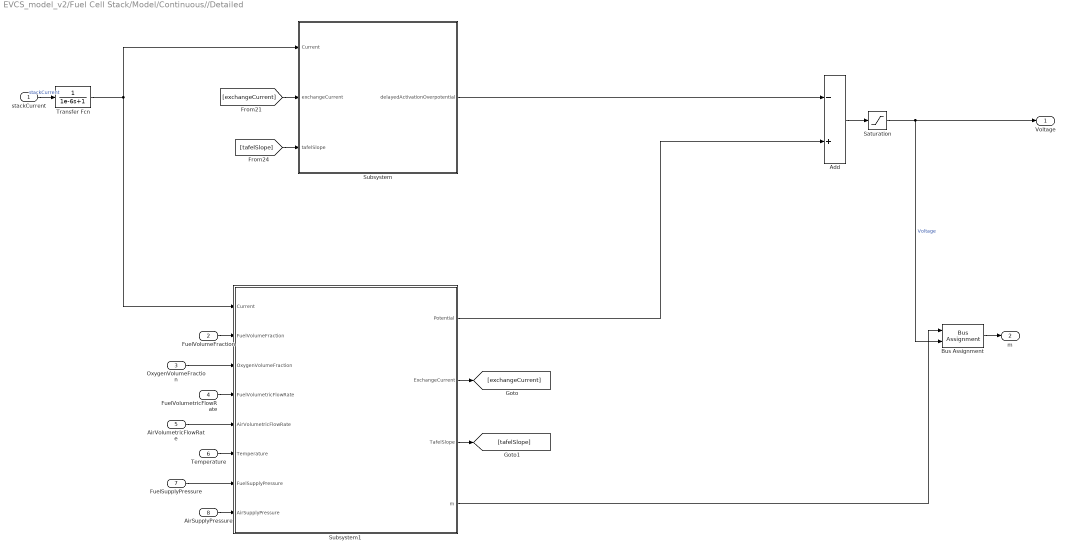
== system EVCS_model_v2/Fuel Cell Stack/Model/Continuous//Detailed ==
  stackCurrent : Inport
  FuelVolumeFraction : Inport  Port=2
  OxygenVolumeFraction : Inport  Port=3
  FuelVolumetricFlowRate : Inport  Port=4
  AirVolumetricFlowRate : Inport  Port=5
  Temperature : Inport  Port=6
  FuelSupplyPressure : Inport  Port=7
  AirSupplyPressure : Inport  Port=8
  Add : Sum  Inputs=-+
  Bus Assignment : BusAssignment  AssignedSignals=Voltage
  Saturation : Saturate  UpperLimit=FC.OCV  LowerLimit=0
  Subsystem : Subsystem
  Subsystem1 : Subsystem
  Transfer Fcn : TransferFcn  Denominator=[1e-6 1]
  Voltage : Outport
  m : Outport  Port=2
  wires:
  Saturation/1 -> Bus Assignment/2, Voltage/1  "Voltage"
  Bus Assignment/1 -> m/1
  stackCurrent/1 -> Transfer Fcn/1  "stackCurrent"
  AirSupplyPressure/1 -> Subsystem1/8(AirSupplyPressure)
  Add/1 -> Saturation/1
  Transfer Fcn/1 -> Subsystem/1(Current), Subsystem1/1(Current)
  AirVolumetricFlowRate/1 -> Subsystem1/5(AirVolumetricFlowRate)
  Subsystem1/2(ExchangeCurrent) -> [exchangeCurrent]
  [exchangeCurrent] -> Subsystem/2(exchangeCurrent)
  FuelSupplyPressure/1 -> Subsystem1/7(FuelSupplyPressure)
  Subsystem1/1(Potential) -> Add/2
  [tafelSlope] -> Subsystem/3(tafelSlope)
  Subsystem1/4(m) -> Bus Assignment/1
  OxygenVolumeFraction/1 -> Subsystem1/3(OxygenVolumeFraction)
  Temperature/1 -> Subsystem1/6(Temperature)
  Subsystem/1(delayedActivationOverpotential) -> Add/1
  FuelVolumeFraction/1 -> Subsystem1/2(FuelVolumeFraction)
  FuelVolumetricFlowRate/1 -> Subsystem1/4(FuelVolumetricFlowRate)
  Subsystem1/3(TafelSlope) -> [tafelSlope]

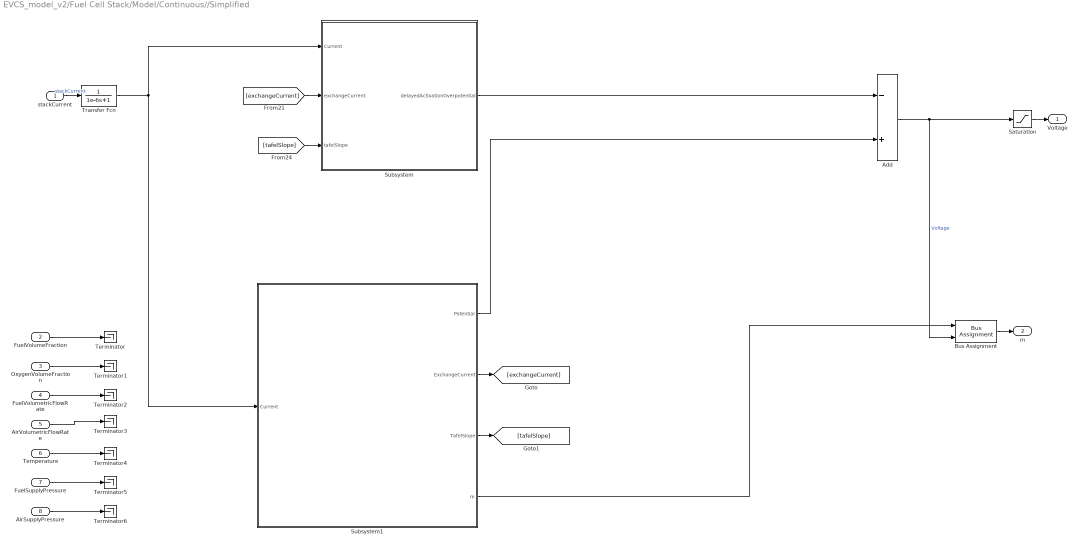
== system EVCS_model_v2/Fuel Cell Stack/Model/Continuous//Simplified ==
  stackCurrent : Inport
  FuelVolumeFraction : Inport  Port=2
  OxygenVolumeFraction : Inport  Port=3
  FuelVolumetricFlowRate : Inport  Port=4
  AirVolumetricFlowRate : Inport  Port=5
  Temperature : Inport  Port=6
  FuelSupplyPressure : Inport  Port=7
  AirSupplyPressure : Inport  Port=8
  Add : Sum  Inputs=-+
  Bus Assignment : BusAssignment  AssignedSignals=Voltage
  Saturation : Saturate  UpperLimit=FC.OCV  LowerLimit=0
  Subsystem : Subsystem
  Subsystem1 : Subsystem
  Terminator{,1..6} (7 alike) : Terminator
  Transfer Fcn : TransferFcn  Denominator=[1e-6 1]
  Voltage : Outport
  m : Outport  Port=2
  wires:
  AirSupplyPressure/1 -> Terminator6/1
  FuelSupplyPressure/1 -> Terminator5/1
  Temperature/1 -> Terminator4/1
  AirVolumetricFlowRate/1 -> Terminator3/1
  FuelVolumetricFlowRate/1 -> Terminator2/1
  OxygenVolumeFraction/1 -> Terminator1/1
  FuelVolumeFraction/1 -> Terminator/1
  Subsystem1/3(TafelSlope) -> [tafelSlope]
  Subsystem1/2(ExchangeCurrent) -> [exchangeCurrent]
  Subsystem1/1(Potential) -> Add/2
  Subsystem/1(delayedActivationOverpotential) -> Add/1
  Subsystem1/4(m) -> Bus Assignment/1
  Saturation/1 -> Voltage/1
  [tafelSlope] -> Subsystem/3(tafelSlope)
  [exchangeCurrent] -> Subsystem/2(exchangeCurrent)
  Transfer Fcn/1 -> Subsystem/1(Current), Subsystem1/1(Current)
  Add/1 -> Saturation/1, Bus Assignment/2  "Voltage"
  stackCurrent/1 -> Transfer Fcn/1  "stackCurrent"
  Bus Assignment/1 -> m/1

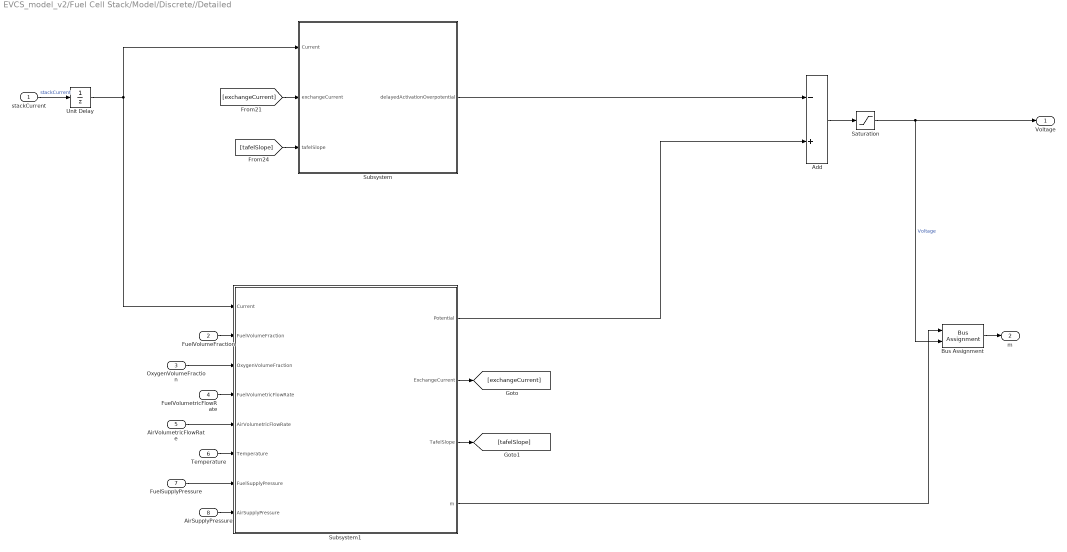
== system EVCS_model_v2/Fuel Cell Stack/Model/Discrete//Detailed ==
  stackCurrent : Inport
  FuelVolumeFraction : Inport  Port=2
  OxygenVolumeFraction : Inport  Port=3
  FuelVolumetricFlowRate : Inport  Port=4
  AirVolumetricFlowRate : Inport  Port=5
  Temperature : Inport  Port=6
  FuelSupplyPressure : Inport  Port=7
  AirSupplyPressure : Inport  Port=8
  Add : Sum  Inputs=-+
  Bus Assignment : BusAssignment  AssignedSignals=Voltage
  Saturation : Saturate  UpperLimit=FC.OCV  LowerLimit=0
  Subsystem : Subsystem
  Subsystem1 : Subsystem
  Unit Delay : UnitDelay  SampleTime=-1  HasFrameUpgradeWarning=on
  Voltage : Outport
  m : Outport  Port=2
  wires:
  Saturation/1 -> Bus Assignment/2, Voltage/1  "Voltage"
  Subsystem1/3(TafelSlope) -> [tafelSlope]
  FuelVolumetricFlowRate/1 -> Subsystem1/4(FuelVolumetricFlowRate)
  FuelVolumeFraction/1 -> Subsystem1/2(FuelVolumeFraction)
  OxygenVolumeFraction/1 -> Subsystem1/3(OxygenVolumeFraction)
  Subsystem1/2(ExchangeCurrent) -> [exchangeCurrent]
  AirVolumetricFlowRate/1 -> Subsystem1/5(AirVolumetricFlowRate)
  Subsystem1/1(Potential) -> Add/2
  FuelSupplyPressure/1 -> Subsystem1/7(FuelSupplyPressure)
  AirSupplyPressure/1 -> Subsystem1/8(AirSupplyPressure)
  Subsystem/1(delayedActivationOverpotential) -> Add/1
  Temperature/1 -> Subsystem1/6(Temperature)
  Subsystem1/4(m) -> Bus Assignment/1
  [tafelSlope] -> Subsystem/3(tafelSlope)
  [exchangeCurrent] -> Subsystem/2(exchangeCurrent)
  Unit Delay/1 -> Subsystem/1(Current), Subsystem1/1(Current)
  Add/1 -> Saturation/1
  stackCurrent/1 -> Unit Delay/1  "stackCurrent"
  Bus Assignment/1 -> m/1

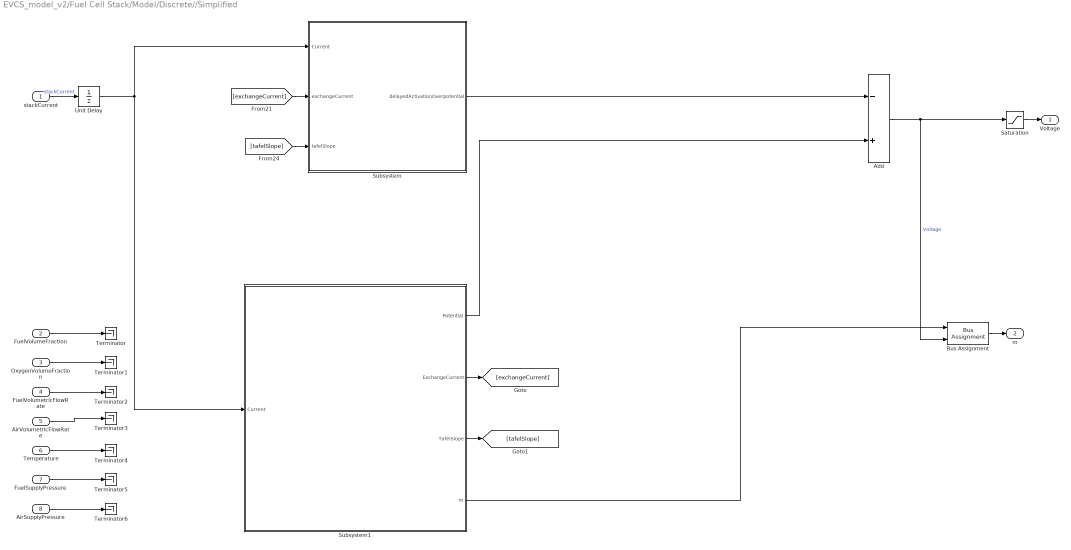
== system EVCS_model_v2/Fuel Cell Stack/Model/Discrete//Simplified ==
  stackCurrent : Inport
  FuelVolumeFraction : Inport  Port=2
  OxygenVolumeFraction : Inport  Port=3
  FuelVolumetricFlowRate : Inport  Port=4
  AirVolumetricFlowRate : Inport  Port=5
  Temperature : Inport  Port=6
  FuelSupplyPressure : Inport  Port=7
  AirSupplyPressure : Inport  Port=8
  Add : Sum  Inputs=-+
  Bus Assignment : BusAssignment  AssignedSignals=Voltage
  Saturation : Saturate  UpperLimit=FC.OCV  LowerLimit=0
  Subsystem : Subsystem
  Subsystem1 : Subsystem
  Terminator{,1..6} (7 alike) : Terminator
  Unit Delay : UnitDelay  SampleTime=-1  HasFrameUpgradeWarning=on
  Voltage : Outport
  m : Outport  Port=2
  wires:
  AirVolumetricFlowRate/1 -> Terminator3/1
  FuelVolumetricFlowRate/1 -> Terminator2/1
  FuelSupplyPressure/1 -> Terminator5/1
  AirSupplyPressure/1 -> Terminator6/1
  Temperature/1 -> Terminator4/1
  OxygenVolumeFraction/1 -> Terminator1/1
  FuelVolumeFraction/1 -> Terminator/1
  Subsystem1/3(TafelSlope) -> [tafelSlope]
  Subsystem1/2(ExchangeCurrent) -> [exchangeCurrent]
  Subsystem1/1(Potential) -> Add/2
  Subsystem/1(delayedActivationOverpotential) -> Add/1
  Subsystem1/4(m) -> Bus Assignment/1
  Saturation/1 -> Voltage/1
  [tafelSlope] -> Subsystem/3(tafelSlope)
  [exchangeCurrent] -> Subsystem/2(exchangeCurrent)
  Unit Delay/1 -> Subsystem/1(Current), Subsystem1/1(Current)
  Add/1 -> Saturation/1, Bus Assignment/2  "Voltage"
  stackCurrent/1 -> Unit Delay/1  "stackCurrent"
  Bus Assignment/1 -> m/1

== system EVCS_model_v2/Fuel Cell Stack/Model/Continuous//Detailed/Subsystem ==
  Current : Inport
  exchangeCurrent : Inport  Port=2
  tafelSlope : Inport  Port=3
  Constant : Constant  Value=1e-9
  Divide : Product  Inputs=*/
  Gain : Gain  Gain=FC.Nc
  Low-Pass Filter (Discrete or Continuous) : eeGeneralControl/Low-Pass Filter (Discrete or Continuous)  K=1  T=FC.Tau  B=inf  A=-inf  init_option=Specify as parameter  x0=0  Ts=Ts
  Math Function : Math  Operator=log
  Product : Product
  Saturation : Saturate  UpperLimit=inf  LowerLimit=0
  Sum : Sum  Inputs=++|
  delayedActivationOverpotential : Outport
  wires:
  Current/1 -> Sum/2
  Gain/1 -> Product/2
  Constant/1 -> Sum/1
  tafelSlope/1 -> Gain/1
  Saturation/1 -> delayedActivationOverpotential/1
  Product/1 -> Low-Pass Filter (Discrete or Continuous)/1
  Sum/1 -> Divide/1
  Divide/1 -> Math Function/1
  Math Function/1 -> Product/1
  Low-Pass Filter (Discrete or Continuous)/1 -> Saturation/1
  exchangeCurrent/1 -> Divide/2
